simulink model "comunicacionArduinoMatlab"  (R2022a)
settings: Solver=VariableStepAuto  StartTime=0.0  StopTime=50  RelTol=1e-3
undefined symbols (not defined in the file): LF
libraries: instrumentseriallib x3, svdutilitieslib x1
settings Model: Creator=felip  LastModifiedBy=felip

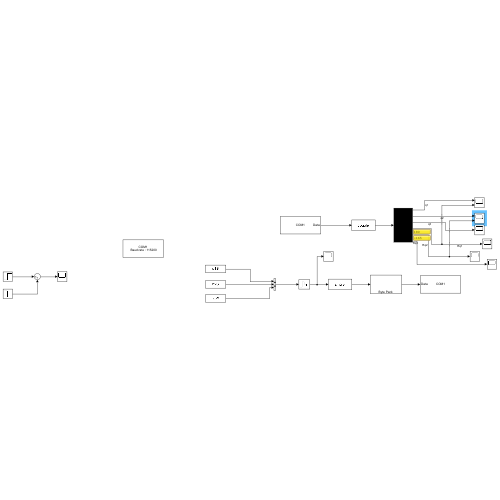
[thumbnail: Simulink's stored preview of the top-level diagram]
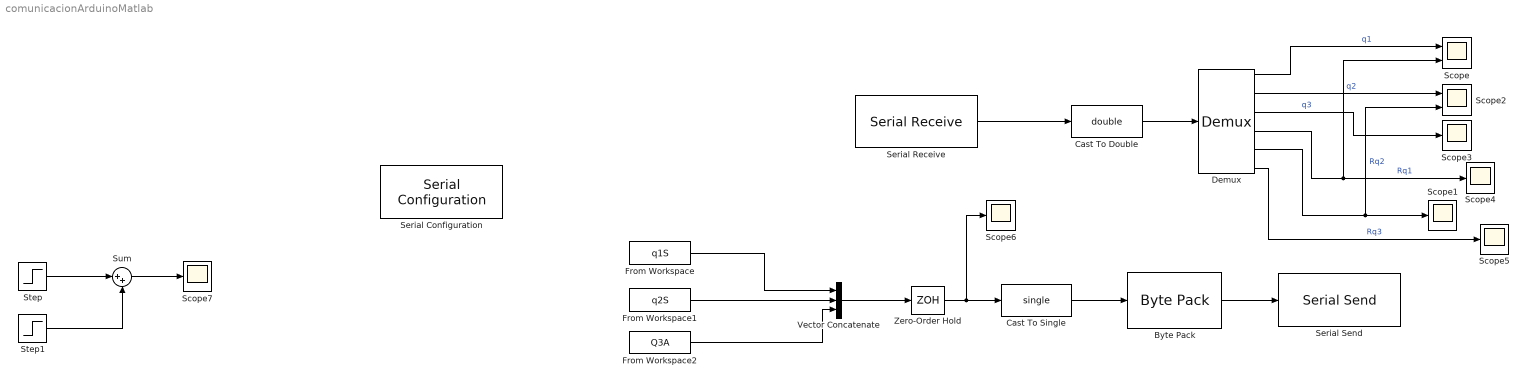
== system comunicacionArduinoMatlab ==
  Byte Pack : svdutilitieslib/Byte Pack  maskPackedDataType=uint32  datatypes={'single'}  byteAlign=4  blockPlatform=arduinoert
      settings: SourceProductBaseCode=ANDROID,ARDUINO,ML_ARDUINO,ECCORTEXA,ECCORTEXR,SC_BEAGLEBONE_BLUE,EC_FREEDOM_BOARD,EC_FRDM_K64F,INTEL_BLOCKSET,MICROBIT,NUCLEO,NVIDIA,PX4AUTOPILOTS,RASPPIIO,STMICRODIS,TIC2000,XILINX_BLOCKSET
  Cast To Double : DataTypeConversion  OutDataTypeStr=double  SaturateOnIntegerOverflow=off  RndMeth=Floor
  Cast To Single : DataTypeConversion  OutDataTypeStr=single  SaturateOnIntegerOverflow=off  RndMeth=Floor
  Demux : Demux  Outputs=6
  From Workspace : FromWorkspace  VariableName=q1S
  From Workspace1 : FromWorkspace  VariableName=q2S
  From Workspace2 : FromWorkspace  VariableName=Q3A
  Scope : Scope  NumInputPorts=2
  Scope{1,3..7} (6 alike) : Scope
  Scope2 : Scope  NumInputPorts=2
  Serial Configuration : instrumentseriallib/Serial Configuration  Priority=-200000  PortSel=COM1  Port=COM1  ComPort=COM1  BaudRate=115200  DataBits=8  Parity=none  StopBits=1  ByteOrder=little-endian  FlowControl=none  Timeout=10  SimulateUsing=Interpreted execution  BlockInModel=on  aMode=1
      settings: SourceProductBaseCode=OT,IC,MT
  Serial Receive : instrumentseriallib/Serial Receive  Priority=1  PortSel=COM1  Port=COM1  ComPort=COM1  DataType=single  SaveDataType=uint8  ToggleHeader=on  Header='A'  ToggleTerminator=on  Terminator=LF ('\n')  CustomTerminator=[]  InputFormat=Column major  ToggleDataSize=on  DataSize=[1 6]  EnableBlockingMode=on  ActionDataUnavailable=Output last received value  ActionWhenDataUnavailable=Output last received value  CustomValue=0  SampleTime=0.005  SimulateUsing=Interpreted execution  BlockInModel=on  aMode=1
      settings: SourceProductBaseCode=OT,IC,MT
  Serial Send : instrumentseriallib/Serial Send  Priority=1  PortSel=COM1  Port=COM1  ComPort=COM1  Header='R'  Terminator=LF ('\n')  CustomTerminator=[]  EnableBlockingMode=on  SimulateUsing=Interpreted execution  BlockInModel=on  aMode=1
      settings: SourceProductBaseCode=OT,IC,MT
  Step : Step  Time=0  After=165  SampleTime=0
  Step1 : Step  Time=5  After=-15  SampleTime=0
  Sum : Sum  Inputs=|++
  Vector Concatenate : Concatenate  NumInputs=3
  Zero-Order Hold : ZeroOrderHold  SampleTime=0.005
  wires:
  Serial Receive/1 -> Cast To Double/1
  Zero-Order Hold/1 -> Scope6/1, Cast To Single/1
  Cast To Single/1 -> Byte Pack/1
  Byte Pack/1 -> Serial Send/1
  Vector Concatenate/1 -> Zero-Order Hold/1
  Demux/1 -> Scope/1  "q1"
  Demux/5 -> Scope2/2, Scope1/1  "Rq2"
  Demux/2 -> Scope2/1  "q2"
  From Workspace1/1 -> Vector Concatenate/2
  From Workspace2/1 -> Vector Concatenate/3
  Demux/3 -> Scope3/1  "q3"
  Demux/4 -> Scope/2, Scope4/1  "Rq1"
  Demux/6 -> Scope5/1  "Rq3"
  Cast To Double/1 -> Demux/1
  Step/1 -> Sum/1
  Step1/1 -> Sum/2
  Sum/1 -> Scope7/1
  From Workspace/1 -> Vector Concatenate/1
